simulink model "AM_Modulation (2)"  (R2023b)
settings: Solver=VariableStepAuto  StartTime=0.0  StopTime=0.01  RelTol=1e-3
settings Model: Creator=ASUS  LastModifiedBy=mahil

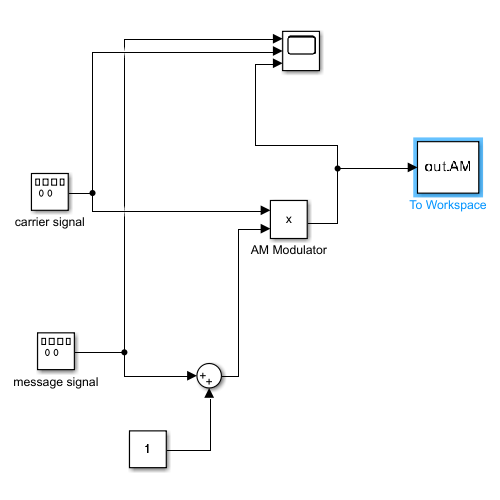
[thumbnail: Simulink's stored preview of the top-level diagram]
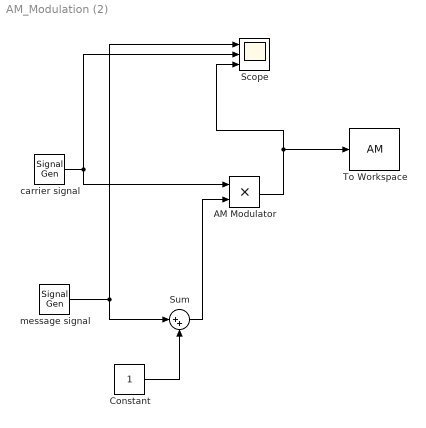
== system AM_Modulation (2) ==
  AM Modulator : Product
  Constant : Constant
  Scope : Scope  NumInputPorts=3
  Sum : Sum  Inputs=|++
  To Workspace : ToWorkspace  VariableName=AM  SampleTime=-1
      settings: Save2DSignal=2-D array (concatenate along first dimension)
  carrier signal : SignalGenerator  Frequency=100000000
  message signal : SignalGenerator  Amplitude=0.5  Frequency=1000
  wires:
  carrier signal/1 -> Scope/2, AM Modulator/1
  message signal/1 -> Sum/1, Scope/1
  AM Modulator/1 -> To Workspace/1, Scope/3
  Constant/1 -> Sum/2
  Sum/1 -> AM Modulator/2
